simulink model "DigitalChannel"  (R2023a)
settings: Solver=VariableStepAuto  StartTime=0.0  StopTime=100  RelTol=1e-3
libraries: commchan3 x1, commrandsrc3 x1, dspfdesign x1, commsink2 x1, dspsigops x1
settings Model: Creator=PANKAJA  LastModifiedBy=PANKAJA

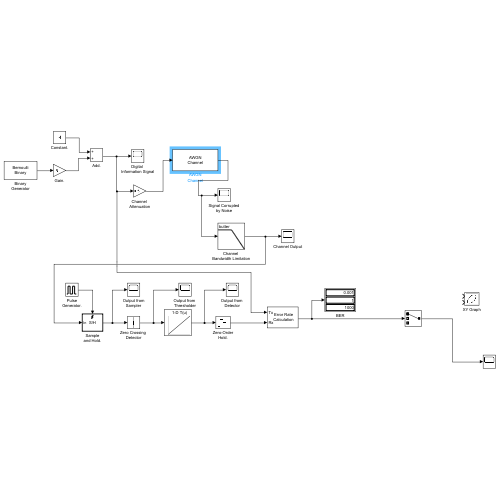
[thumbnail: Simulink's stored preview of the top-level diagram]
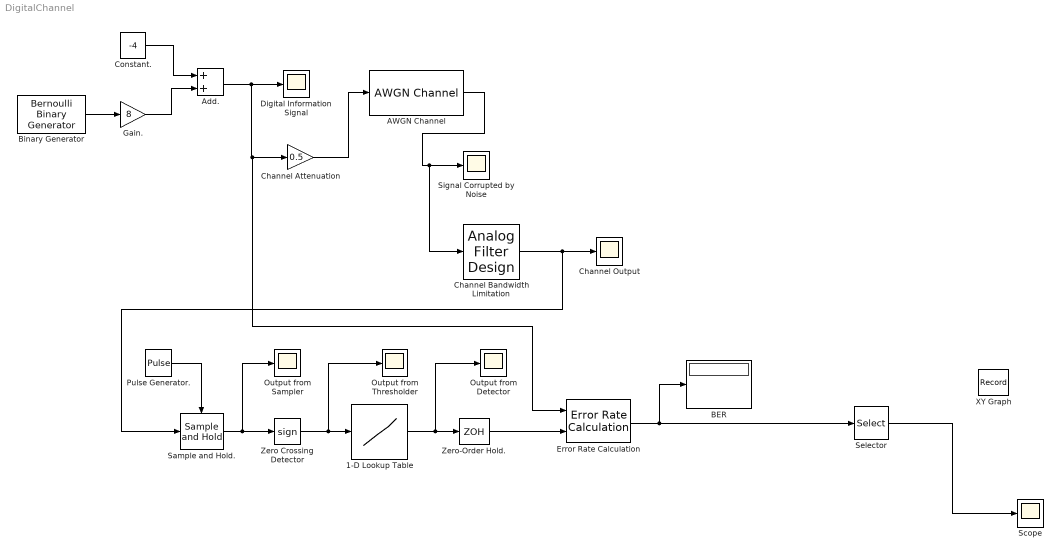
== system DigitalChannel ==
  1-D Lookup Table : Lookup_n-D  NumberOfTableDimensions=1  BreakpointsForDimension1=[-1,1]  Table=[-4,4]  InternalRulePriority=Speed  RndMeth=Simplest
  AWGN Channel : commchan3/AWGN Channel  LegacyMode=off  NoiseMethod="Signal to noise ratio  (SNR)"  noiseMode="Signal to noise ratio  (SNR)"  EbNo=3  EsNo=10  SNR=4  BitsPerSymbol=1  SignalPower=1  SamplesPerSymbol=1  SymbolPeriod=1  VarianceSource=Parameter  Variance=1  RandomStream=Global stream  Seed=67  SimulateUsing=Code generation
  Add. : Sum
  BER : Display
  Binary Generator : commrandsrc3/Bernoulli Binary Generator  ProbabilityOfZero=0.5  SeedSource=Parameter  Seed=61  SampleTime=0.1  SamplesPerFrame=1  OutputDataType=double  SimulateUsing=Interpreted execution
  Channel Attenuation : Gain  Gain=0.5
  Channel Bandwidth Limitation : dspfdesign/Analog Filter Design  method=Butterworth  filttype=Lowpass  N=10  Wlo=1000  Whi=80  Rp=2  Rs=40
  Channel Output : Scope
  Constant. : Constant  Value=-4
  Digital Information Signal : Scope
  Error Rate Calculation : commsink2/Error Rate Calculation  N=1  st_delay=0  cp_mode=Entire frame  subframe=[]  PMode=Port  WsName=ErrorVec  RsMode2=off  stop=off  numErr=100  maxBits=1e6
  Gain. : Gain  Gain=8
  Output from Sampler : Scope
  Output from Detector : Scope
  Output from Thresholder : Scope
  Pulse Generator. : DiscretePulseGenerator  PulseType=Time based  Period=0.1  PulseWidth=50
  Sample and Hold. : dspsigops/Sample and Hold  trig=Rising edge  initCond=0  latchinput=off
  Scope : Scope
  Selector : Selector  InputPortWidth=3  IndexOptions=Index vector (dialog)  Indices=[1]  OutputSizes=1
  Signal Corrupted by Noise : Scope
  XY Graph : Record  FileSettingsInternal="{\"entries\":[{\"content\":{\"excelSettings\":{\"content\":{},\"type\":\"Streamout.ExcelSettings\"}},\"type\":\"Streamout.FileSettingStorage\",\"uuid\":\"fcca9526-da08-4939-8b08-3b77a2af3b0d\"}],\"packageUris\":[\"http://schema.mathworks.com/mf0/streamout_blocks/R2020a\"],\"version\":\"1.0\"}"  Layout=[1 1]  SignalsInternal="{\"entries\":[{\"content\":{\"signals\":[{\"content\":{\"blockPath\":[\"DigitalChannel/XY Graph\"],\"dimensions\":[1],\"domain\":\"DigitalChannel/XY Graph\",\"lineColor\":\"#a2142f\",\"plots\":[1],\"port\":1,\"sid\":[\"\"],\"signalID\":2067},\"type\":\"RecordBlkView.Signal\",\"uuid\":\"8fabe924-985a-4adb-84db-5ec980484a71\"},{\"content\":{\"blockPath\":[\"DigitalChannel/XY Graph\"],\"dimensions\":[1],\"domain\":\"DigitalChannel/XY Graph\",\"lineColor\":\"#139fff\",\"plots\":[1],\"port\":2,\"sid\":[\"\"],\"signalID\":2071},\"type\":\"RecordBlkView.Signal\",\"uuid\":\"e70ba62d-7bb2-4548-88e2-ff924df3405f\"}]},\"type\":\"RecordBlkView.InputSignals\",\"uuid\":\"683bc100-5dbb-40fe-ba77-c2002cdc5ad1\"}],\"packageUris\":[\"http://schema.mathworks.com/mf0/streamout_blocks/R2020a\"],\"version\":\"1.0\"}"  VisualizationBindings="{\"xyplotplugin\":{\"info\":[{\"series\":[{\"bindingParametersList\":[{\"parameter\":\"X-Axis\",\"signalID\":2067,\"signalName\":\"XY Graph:1\"},{\"parameter\":\"Y-Axis\",\"signalID\":2071,\"signalName\":\"XY Graph:2\"}],\"seriesID\":25760}],\"subplotID\":1}]}}"  CompatibilityTag=XY
  Zero Crossing Detector : Signum
  Zero-Order Hold. : ZeroOrderHold  SampleTime=0.1
  wires:
  Binary Generator/1 -> Gain./1
  Constant./1 -> Add./1
  Gain./1 -> Add./2
  Add./1 -> Error Rate Calculation/1, Channel Attenuation/1, Digital Information Signal/1
  AWGN Channel/1 -> Channel Bandwidth Limitation/1, Signal Corrupted by Noise/1
  Pulse Generator./1 -> Sample and Hold./Trigger
  Sample and Hold./1 -> Output from Sampler/1, Zero Crossing Detector/1
  Zero Crossing Detector/1 -> 1-D Lookup Table/1, Output from Thresholder/1
  1-D Lookup Table/1 -> Output from Detector/1, Zero-Order Hold./1
  Zero-Order Hold./1 -> Error Rate Calculation/2
  Error Rate Calculation/1 -> BER/1, Selector/1
  Channel Bandwidth Limitation/1 -> Sample and Hold./1, Channel Output/1
  Channel Attenuation/1 -> AWGN Channel/1
  Selector/1 -> Scope/1
